simulink model "Robust_design_step_validation_2_1_2_5"  (R2024b)
settings: Solver=ode5  StartTime=0.0  StopTime=10  FixedStep=10e-06  RelTol=1e-3
undefined symbols (not defined in the file): Ao, Bo, Co, daq, Do, drv, gbox, index, K_vec, mld, mot, Nu, Nx, rpm2rads, sens, step_gain, T, Ts, u_bar_max
settings Model: Creator=Enrico  LastModifiedBy=farin
settings DataIOCC: ReturnWorkspaceOutputsName=out_black_box

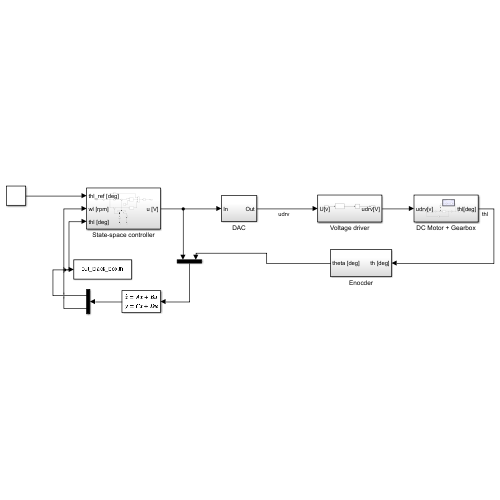
[thumbnail: Simulink's stored preview of the top-level diagram]
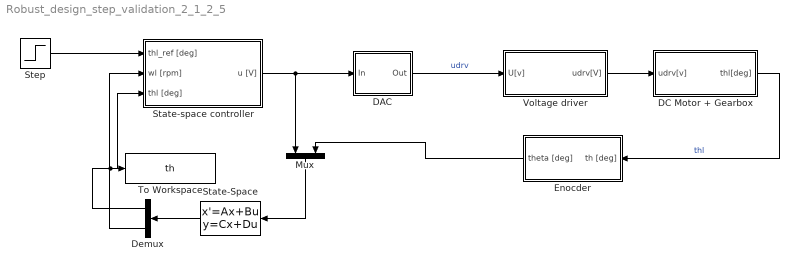
== system Robust_design_step_validation_2_1_2_5 ==
  DAC : Subsystem
  DC Motor + Gearbox : Subsystem
  Demux : Demux  Outputs=2
  Enocder : Subsystem
  Mux : Mux  Inputs=2
  State-Space : StateSpace  A=Ao  B=Bo  C=Co  D=Do  InitialCondition=0
  State-space controller : Subsystem
  Step : Step  After=step_gain  SampleTime=0
  To Workspace : ToWorkspace  VariableName=th  SaveFormat=Structure With Time  SampleTime=-1
  Voltage driver : Subsystem
  wires:
  DAC/1(Out) -> Voltage driver/1(U[v])  "udrv"
  Voltage driver/1(udrv[V]) -> DC Motor + Gearbox/1(udrv[v])
  Mux/1 -> State-Space/1
  State-Space/1 -> Demux/1
  Demux/1 -> State-space controller/3(thl [deg]), To Workspace/1
  Enocder/1(theta [deg]) -> Mux/2
  DC Motor + Gearbox/1(thl[deg]) -> Enocder/1(th [deg])  "thl"
  Step/1 -> State-space controller/1(thl_ref [deg])
  Demux/2 -> State-space controller/2(wl [rpm])
  State-space controller/1(u [V]) -> Mux/1, DAC/1(In)

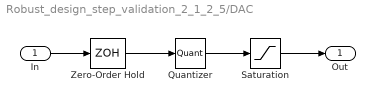
== system Robust_design_step_validation_2_1_2_5/DAC ==
  In : Inport
  Quantizer : Quantizer  QuantizationInterval=daq.dac.q
  Saturation : Saturate  UpperLimit=daq.dac.fs  LowerLimit=-daq.dac.fs
  Zero-Order Hold : ZeroOrderHold  SampleTime=Ts
  Out : Outport
  wires:
  Quantizer/1 -> Saturation/1
  In/1 -> Zero-Order Hold/1
  Zero-Order Hold/1 -> Quantizer/1
  Saturation/1 -> Out/1

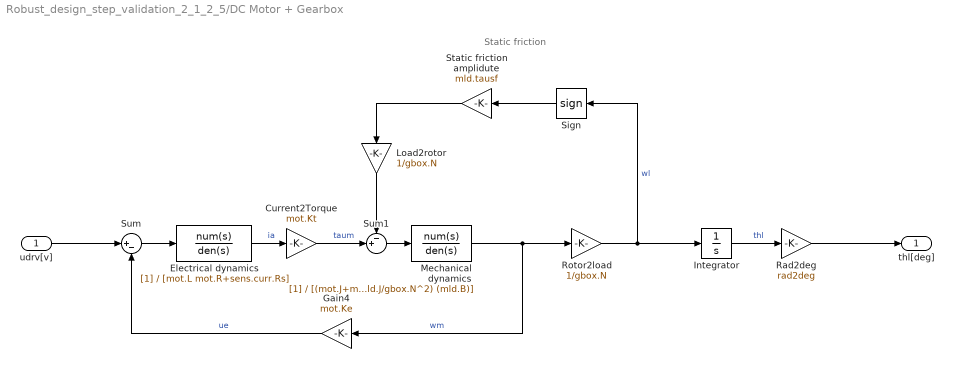
== system Robust_design_step_validation_2_1_2_5/DC Motor + Gearbox ==
  note: Static friction
  udrv[v] : Inport
  " Sign" : Signum  ZeroCross=off
  Current2Torque : Gain  Gain=mot.Kt
  Electrical dynamics : TransferFcn  Denominator=[mot.L mot.R+sens.curr.Rs]
  Gain4 : Gain  Gain=mot.Ke
  Integrator : Integrator
  Load2rotor : Gain  Gain=1/gbox.N
  Mechanical dynamics : TransferFcn  Denominator=[(mot.J+mld.J/gbox.N^2) (mld.B)]
  Rad2deg : Gain  Gain=rad2deg
  Rotor2load : Gain  Gain=1/gbox.N
  Static friction amplidute : Gain  Gain=mld.tausf
  Sum : Sum  Inputs=|+-
  Sum1 : Sum  Inputs=-+|
  thl[deg] : Outport
  wires:
  udrv[v]/1 -> Sum/1
  Sum/1 -> Electrical dynamics/1
  Electrical dynamics/1 -> Current2Torque/1  "ia"
  Current2Torque/1 -> Sum1/2  "taum"
  Load2rotor/1 -> Sum1/1
  " Sign"/1 -> Static friction amplidute/1
  Static friction amplidute/1 -> Load2rotor/1
  Sum1/1 -> Mechanical dynamics/1
  Mechanical dynamics/1 -> Gain4/1, Rotor2load/1  "wm"
  Gain4/1 -> Sum/2  "ue"
  Rad2deg/1 -> thl[deg]/1
  Integrator/1 -> Rad2deg/1  "thl"
  Rotor2load/1 -> " Sign"/1, Integrator/1  "wl"

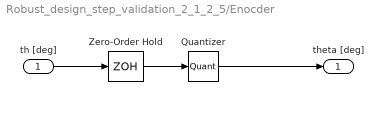
== system Robust_design_step_validation_2_1_2_5/Enocder ==
  th [deg] : Inport
  Quantizer : Quantizer  QuantizationInterval=sens.enc.pulse2deg
  Zero-Order Hold : ZeroOrderHold  SampleTime=T
  theta [deg] : Outport
  wires:
  th [deg]/1 -> Zero-Order Hold/1
  Zero-Order Hold/1 -> Quantizer/1
  Quantizer/1 -> theta [deg]/1

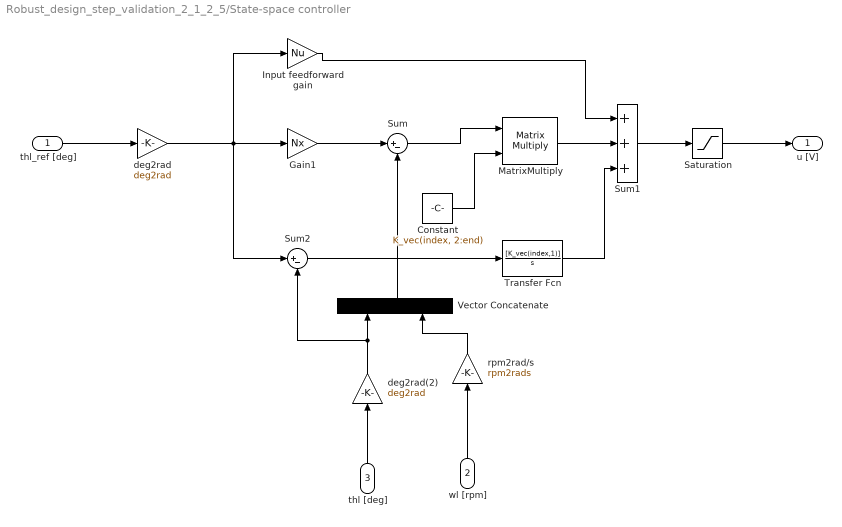
== system Robust_design_step_validation_2_1_2_5/State-space controller ==
  thl_ref [deg] : Inport
  wl [rpm] : Inport  Port=2
  thl [deg] : Inport  Port=3
  Constant : Constant  Value=K_vec(index, 2:end)
  Gain1 : Gain  Gain=Nx
  Input feedforward gain : Gain  Gain=Nu
  MatrixMultiply : Product  Multiplication=Matrix(*)
  Saturation : Saturate  UpperLimit=u_bar_max  LowerLimit=-u_bar_max
  Sum : Sum  Inputs=|+-
  Sum1 : Sum  Inputs=+++
  Sum2 : Sum  Inputs=|+-
  Transfer Fcn : TransferFcn  Numerator=[K_vec(index,1)]  Denominator=[1 0]
  Vector Concatenate : Concatenate
  deg2rad : Gain  Gain=deg2rad
  deg2rad(2) : Gain  Gain=deg2rad
  rpm2rad/s : Gain  Gain=rpm2rads
  u [V] : Outport
  wires:
  Sum2/1 -> Transfer Fcn/1
  deg2rad(2)/1 -> Vector Concatenate/1, Sum2/2
  Constant/1 -> MatrixMultiply/2
  thl_ref [deg]/1 -> deg2rad/1
  Input feedforward gain/1 -> Sum1/1
  Saturation/1 -> u [V]/1
  MatrixMultiply/1 -> Sum1/2
  Transfer Fcn/1 -> Sum1/3
  Sum/1 -> MatrixMultiply/1
  wl [rpm]/1 -> rpm2rad/s/1
  Vector Concatenate/1 -> Sum/2
  thl [deg]/1 -> deg2rad(2)/1
  deg2rad/1 -> Gain1/1, Sum2/1, Input feedforward gain/1
  rpm2rad/s/1 -> Vector Concatenate/2
  Gain1/1 -> Sum/1
  Sum1/1 -> Saturation/1

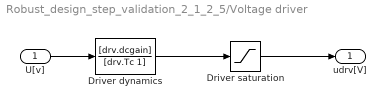
== system Robust_design_step_validation_2_1_2_5/Voltage driver ==
  U[v] : Inport
  Driver dynamics : TransferFcn  Numerator=[drv.dcgain]  Denominator=[drv.Tc 1]
  Driver saturation : Saturate  UpperLimit=12  LowerLimit=-12
  udrv[V] : Outport
  wires:
  U[v]/1 -> Driver dynamics/1
  Driver dynamics/1 -> Driver saturation/1
  Driver saturation/1 -> udrv[V]/1
